simulink model "(1) DePatieFinalSimulation_NDEPA"  (R2021a)
settings: Solver=VariableStepAuto  StartTime=0.0  StopTime=400  RelTol=1e-3
libraries: simulink x1
settings Model: Creator=nwdep  LastModifiedBy=nwdep
settings SolverCC: ZeroCrossAlgorithm=Adaptive

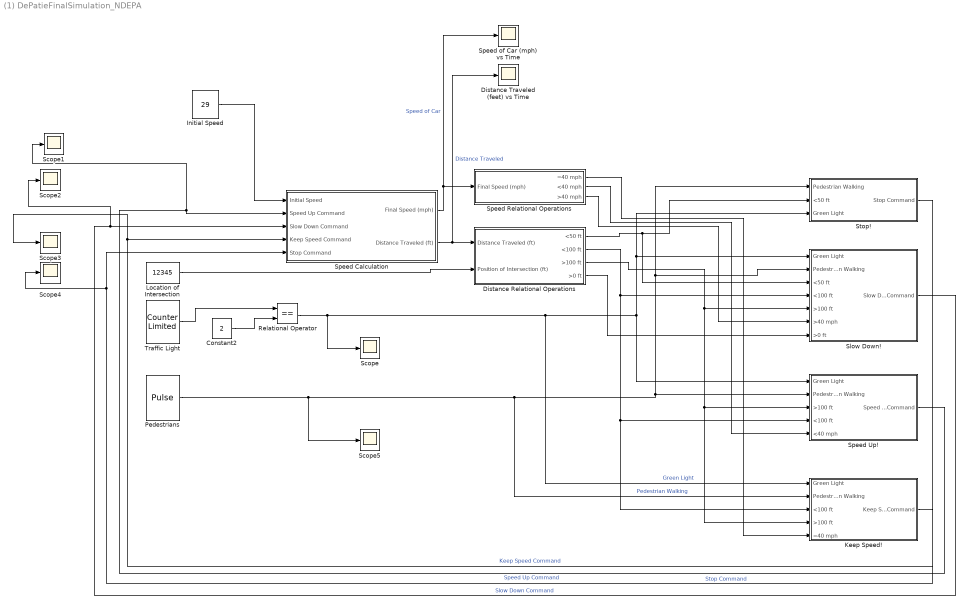
== system (1) DePatieFinalSimulation_NDEPA ==
  Constant2 : Constant  Value=2
  Distance Relational Operations : Subsystem
  Distance Traveled (feet) vs Time : Scope
  Initial Speed : Constant  Value=29
  Keep Speed! : Subsystem
  Location of Intersection : Constant  Value=12345
  Pedestrians : DiscretePulseGenerator  PulseType=Time based  Period=30  PulseWidth=50
  Relational Operator : RelationalOperator  Operator===  OutDataTypeStr=boolean  RndMeth=Simplest
  Scope{,1..5} (6 alike) : Scope
  Slow Down! : Subsystem
  Speed Calculation : Subsystem
  Speed Relational Operations : Subsystem
  Speed Up! : Subsystem
  Speed of Car (mph) vs Time : Scope
  Stop! : Subsystem
  Traffic Light : simulink/Sources/Counter Limited  uplimit=2  tsamp=60
  wires:
  Initial Speed/1 -> Speed Calculation/1(Initial Speed)
  Traffic Light/1 -> Relational Operator/1
  Constant2/1 -> Relational Operator/2
  Relational Operator/1 -> Scope/1, Keep Speed!/1(Green Light), Speed Up!/1(Green Light), Stop!/3(Green Light), Slow Down!/1(Green Light)  "Green Light"
  Pedestrians/1 -> Scope5/1, Keep Speed!/2(Pedestrian Walking), Stop!/1(Pedestrian Walking), Slow Down!/2(Pedestrian Walking), Speed Up!/2(Pedestrian Walking)  "Pedestrian Walking"
  Speed Calculation/1(Final Speed (mph)) -> Speed of Car (mph) vs Time/1, Speed Relational Operations/1(Final Speed (mph))  "Speed of Car"
  Speed Calculation/2(Distance Traveled (ft)) -> Distance Traveled (feet) vs Time/1, Distance Relational Operations/1(Distance Traveled (ft))  "Distance Traveled"
  Distance Relational Operations/1(<50 ft) -> Stop!/2(<50 ft), Slow Down!/3(<50 ft)
  Distance Relational Operations/2(<100 ft) -> Keep Speed!/3(<100 ft), Speed Up!/4(<100 ft), Slow Down!/4(<100 ft)
  Distance Relational Operations/3(>100 ft) -> Keep Speed!/4(>100 ft), Speed Up!/3(>100 ft), Slow Down!/5(>100 ft)
  Speed Relational Operations/3(>40 mph) -> Slow Down!/6(>40 mph)
  Speed Relational Operations/2(<40 mph) -> Speed Up!/5(<40 mph)
  Location of Intersection/1 -> Distance Relational Operations/2(Position of Intersection (ft))
  Speed Relational Operations/1(=40 mph) -> Keep Speed!/5(=40 mph)
  Keep Speed!/1(Keep Speed Command) -> Scope3/1, Speed Calculation/4(Keep Speed Command)  "Keep Speed Command"
  Speed Up!/1(Speed Up Command) -> Scope1/1, Speed Calculation/2(Speed Up Command)  "Speed Up Command"
  Slow Down!/1(Slow Down Command) -> Scope2/1, Speed Calculation/3(Slow Down Command)  "Slow Down Command"
  Stop!/1(Stop Command) -> Scope4/1, Speed Calculation/5(Stop Command)  "Stop Command"
  Distance Relational Operations/4(>0 ft) -> Slow Down!/7(>0 ft)

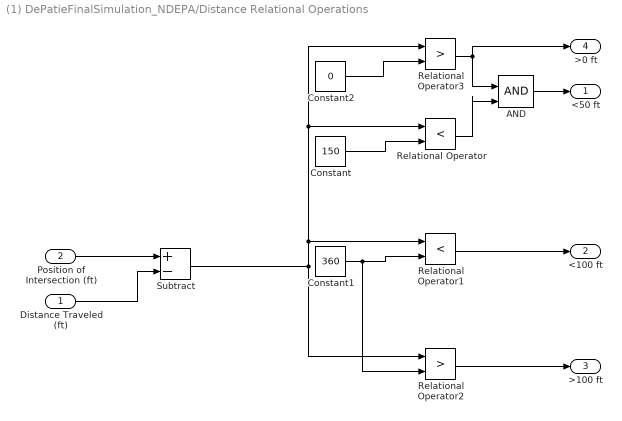
== system (1) DePatieFinalSimulation_NDEPA/Distance Relational Operations ==
  Distance Traveled (ft) : Inport
  Position of Intersection (ft) : Inport  Port=2
  AND : Logic  IconShape=distinctive  AllPortsSameDT=off  OutDataTypeStr=boolean
  Constant : Constant  Value=150
  Constant1 : Constant  Value=360
  Constant2 : Constant  Value=0
  Relational Operator : RelationalOperator  Operator=<  OutDataTypeStr=boolean  RndMeth=Simplest
  Relational Operator1 : RelationalOperator  Operator=<  OutDataTypeStr=boolean  RndMeth=Simplest
  Relational Operator2 : RelationalOperator  Operator=>  OutDataTypeStr=boolean  RndMeth=Simplest
  Relational Operator3 : RelationalOperator  Operator=>  OutDataTypeStr=boolean  RndMeth=Simplest
  Subtract : Sum  Inputs=+-
  <50 ft : Outport
  <100 ft : Outport  Port=2
  >100 ft : Outport  Port=3
  >0 ft : Outport  Port=4
  wires:
  Constant/1 -> Relational Operator/2
  Relational Operator1/1 -> <100 ft/1
  Relational Operator2/1 -> >100 ft/1
  Constant1/1 -> Relational Operator2/2, Relational Operator1/2
  Subtract/1 -> Relational Operator3/1, Relational Operator/1, Relational Operator1/1, Relational Operator2/1
  Position of Intersection (ft)/1 -> Subtract/1
  Distance Traveled (ft)/1 -> Subtract/2
  Constant2/1 -> Relational Operator3/2
  AND/1 -> <50 ft/1
  Relational Operator3/1 -> AND/1, >0 ft/1
  Relational Operator/1 -> AND/2

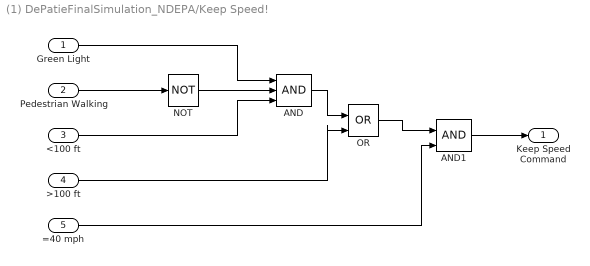
== system (1) DePatieFinalSimulation_NDEPA/Keep Speed! ==
  Green Light : Inport
  Pedestrian Walking : Inport  Port=2
  <100 ft : Inport  Port=3
  >100 ft : Inport  Port=4
  =40 mph : Inport  Port=5
  AND : Logic  Inputs=3  IconShape=distinctive  AllPortsSameDT=off  OutDataTypeStr=boolean
  AND1 : Logic  IconShape=distinctive  AllPortsSameDT=off  OutDataTypeStr=boolean
  NOT : Logic  Operator=NOT  IconShape=distinctive  AllPortsSameDT=off  OutDataTypeStr=boolean
  OR : Logic  Operator=OR  IconShape=distinctive  AllPortsSameDT=off  OutDataTypeStr=boolean
  Keep Speed Command : Outport
  wires:
  Pedestrian Walking/1 -> NOT/1
  Green Light/1 -> AND/1
  NOT/1 -> AND/2
  <100 ft/1 -> AND/3
  >100 ft/1 -> OR/2
  AND/1 -> OR/1
  OR/1 -> AND1/1
  =40 mph/1 -> AND1/2
  AND1/1 -> Keep Speed Command/1

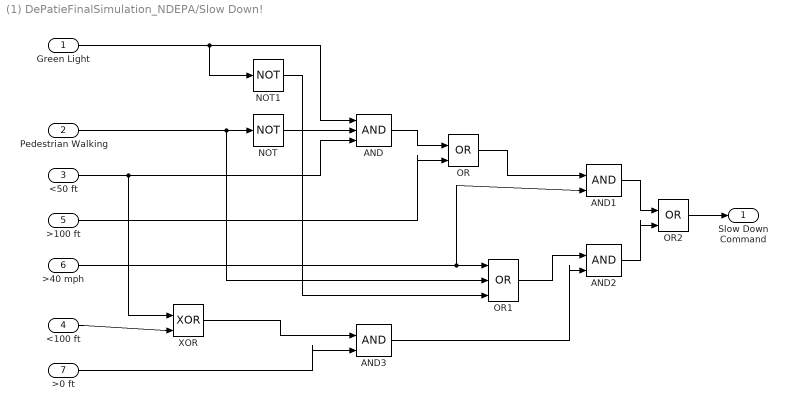
== system (1) DePatieFinalSimulation_NDEPA/Slow Down! ==
  Green Light : Inport
  Pedestrian Walking : Inport  Port=2
  <50 ft : Inport  Port=3
  <100 ft : Inport  Port=4
  >100 ft : Inport  Port=5
  >40 mph : Inport  Port=6
  >0 ft : Inport  Port=7
  AND : Logic  Inputs=3  IconShape=distinctive  AllPortsSameDT=off  OutDataTypeStr=boolean
  AND1 : Logic  IconShape=distinctive  AllPortsSameDT=off  OutDataTypeStr=boolean
  AND2 : Logic  IconShape=distinctive  AllPortsSameDT=off  OutDataTypeStr=boolean
  AND3 : Logic  IconShape=distinctive  AllPortsSameDT=off  OutDataTypeStr=boolean
  NOT : Logic  Operator=NOT  IconShape=distinctive  AllPortsSameDT=off  OutDataTypeStr=boolean
  NOT1 : Logic  Operator=NOT  IconShape=distinctive  AllPortsSameDT=off  OutDataTypeStr=boolean
  OR : Logic  Operator=OR  IconShape=distinctive  AllPortsSameDT=off  OutDataTypeStr=boolean
  OR1 : Logic  Operator=OR  Inputs=3  IconShape=distinctive  AllPortsSameDT=off  OutDataTypeStr=boolean
  OR2 : Logic  Operator=OR  IconShape=distinctive  AllPortsSameDT=off  OutDataTypeStr=boolean
  XOR : Logic  Operator=XOR  IconShape=distinctive  AllPortsSameDT=off  OutDataTypeStr=boolean
  Slow Down Command : Outport
  wires:
  Pedestrian Walking/1 -> OR1/2, NOT/1
  NOT/1 -> AND/2
  AND/1 -> OR/1
  >100 ft/1 -> OR/2
  Green Light/1 -> NOT1/1, AND/1
  <50 ft/1 -> XOR/1, AND/3
  OR/1 -> AND1/1
  >40 mph/1 -> AND1/2, OR1/1
  NOT1/1 -> OR1/3
  OR1/1 -> AND2/1
  AND1/1 -> OR2/1
  AND2/1 -> OR2/2
  OR2/1 -> Slow Down Command/1
  <100 ft/1 -> XOR/2
  XOR/1 -> AND3/1
  >0 ft/1 -> AND3/2
  AND3/1 -> AND2/2

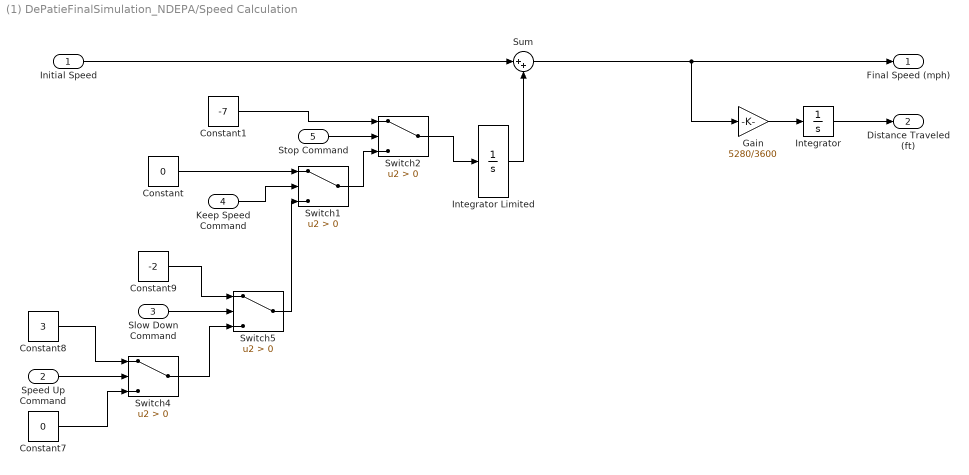
== system (1) DePatieFinalSimulation_NDEPA/Speed Calculation ==
  Initial Speed : Inport
  Speed Up Command : Inport  Port=2
  Slow Down Command : Inport  Port=3
  Keep Speed Command : Inport  Port=4
  Stop Command : Inport  Port=5
  Constant : Constant  Value=0
  Constant1 : Constant  Value=-7
  Constant7 : Constant  Value=0
  Constant8 : Constant  Value=3
  Constant9 : Constant  Value=-2
  Gain : Gain  Gain=5280/3600
  Integrator : Integrator
  Integrator Limited : Integrator  LimitOutput=on  UpperSaturationLimit=70  LowerSaturationLimit=-29
  Sum : Sum  Inputs=|++
  Switch{1..2,4..5} (4 alike) : Switch  Criteria=u2 > Threshold
  Final Speed (mph) : Outport
  Distance Traveled (ft) : Outport  Port=2
  wires:
  Initial Speed/1 -> Sum/1
  Sum/1 -> Gain/1, Final Speed (mph)/1
  Switch4/1 -> Switch5/3
  Constant7/1 -> Switch4/3
  Constant8/1 -> Switch4/1
  Constant9/1 -> Switch5/1
  Integrator Limited/1 -> Sum/2
  Speed Up Command/1 -> Switch4/2
  Slow Down Command/1 -> Switch5/2
  Integrator/1 -> Distance Traveled (ft)/1
  Gain/1 -> Integrator/1
  Keep Speed Command/1 -> Switch1/2
  Switch5/1 -> Switch1/3
  Constant/1 -> Switch1/1
  Switch1/1 -> Switch2/3
  Switch2/1 -> Integrator Limited/1
  Stop Command/1 -> Switch2/2
  Constant1/1 -> Switch2/1

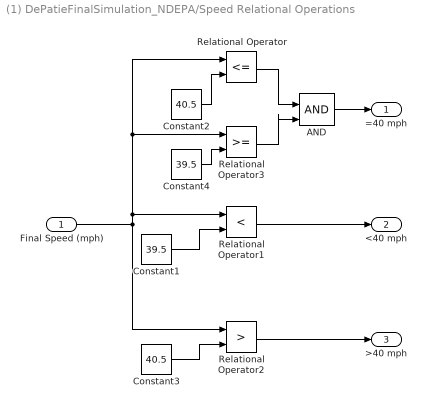
== system (1) DePatieFinalSimulation_NDEPA/Speed Relational Operations ==
  Final Speed (mph) : Inport
  AND : Logic  IconShape=distinctive  AllPortsSameDT=off  OutDataTypeStr=boolean
  Constant1 : Constant  Value=39.5
  Constant2 : Constant  Value=40.5
  Constant3 : Constant  Value=40.5
  Constant4 : Constant  Value=39.5
  Relational Operator : RelationalOperator  Operator=<=  OutDataTypeStr=boolean  RndMeth=Simplest
  Relational Operator1 : RelationalOperator  Operator=<  OutDataTypeStr=boolean  RndMeth=Simplest
  Relational Operator2 : RelationalOperator  Operator=>  OutDataTypeStr=boolean  RndMeth=Simplest
  Relational Operator3 : RelationalOperator  OutDataTypeStr=boolean  RndMeth=Simplest
  =40 mph : Outport
  <40 mph : Outport  Port=2
  >40 mph : Outport  Port=3
  wires:
  Final Speed (mph)/1 -> Relational Operator2/1, Relational Operator/1, Relational Operator3/1, Relational Operator1/1
  Relational Operator1/1 -> <40 mph/1
  Relational Operator2/1 -> >40 mph/1
  Constant3/1 -> Relational Operator2/2
  Constant1/1 -> Relational Operator1/2
  Constant2/1 -> Relational Operator/2
  Relational Operator/1 -> AND/1
  Constant4/1 -> Relational Operator3/2
  AND/1 -> =40 mph/1
  Relational Operator3/1 -> AND/2

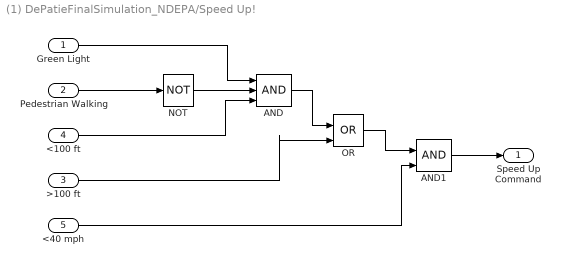
== system (1) DePatieFinalSimulation_NDEPA/Speed Up! ==
  Green Light : Inport
  Pedestrian Walking : Inport  Port=2
  >100 ft : Inport  Port=3
  <100 ft : Inport  Port=4
  <40 mph : Inport  Port=5
  AND : Logic  Inputs=3  IconShape=distinctive  AllPortsSameDT=off  OutDataTypeStr=boolean
  AND1 : Logic  IconShape=distinctive  AllPortsSameDT=off  OutDataTypeStr=boolean
  NOT : Logic  Operator=NOT  IconShape=distinctive  AllPortsSameDT=off  OutDataTypeStr=boolean
  OR : Logic  Operator=OR  IconShape=distinctive  AllPortsSameDT=off  OutDataTypeStr=boolean
  Speed Up Command : Outport
  wires:
  Pedestrian Walking/1 -> NOT/1
  NOT/1 -> AND/2
  Green Light/1 -> AND/1
  <100 ft/1 -> AND/3
  AND/1 -> OR/1
  >100 ft/1 -> OR/2
  OR/1 -> AND1/1
  <40 mph/1 -> AND1/2
  AND1/1 -> Speed Up Command/1

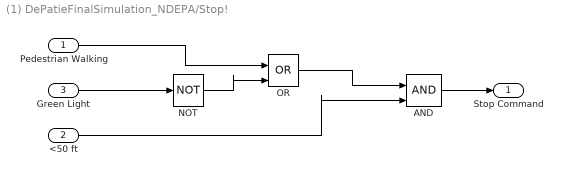
== system (1) DePatieFinalSimulation_NDEPA/Stop! ==
  Pedestrian Walking : Inport
  <50 ft : Inport  Port=2
  Green Light : Inport  Port=3
  AND : Logic  IconShape=distinctive  AllPortsSameDT=off  OutDataTypeStr=boolean
  NOT : Logic  Operator=NOT  IconShape=distinctive  AllPortsSameDT=off  OutDataTypeStr=boolean
  OR : Logic  Operator=OR  IconShape=distinctive  AllPortsSameDT=off  OutDataTypeStr=boolean
  Stop Command : Outport
  wires:
  Green Light/1 -> NOT/1
  NOT/1 -> OR/2
  AND/1 -> Stop Command/1
  <50 ft/1 -> AND/2
  Pedestrian Walking/1 -> OR/1
  OR/1 -> AND/1
